simulink model "a2_clutch_control_sim"  (R2022b)
settings: Solver=VariableStepAuto  StartTime=0.0  StopTime=60  RelTol=1e-3
values from neighbouring files (symbols this model uses):
  Kd = 0.0033    [a1_performance_analysis_PD.m]    (also in a1_performance_analysis_PD_vs_Template.m; a2_hinf_control.m; a2_hinf_control_uncertainties.m)
  Kp = 0.3    [a1_performance_analysis_PD.m]    (also in a1_performance_analysis_PD_vs_Template.m; a2_hinf_control.m; a2_hinf_control_uncertainties.m)
  noise_fre = 800    [a2_hinf_control.m]    (also in a2_hinf_control_uncertainties.m)
undefined symbols (not defined in the file or in its folder): K_inf, vx
libraries: cstblocks x4, slpidlib x1
settings Model: Creator=phatdo  LastModifiedBy=phatdo
settings DataIOCC: ReturnWorkspaceOutputs=off

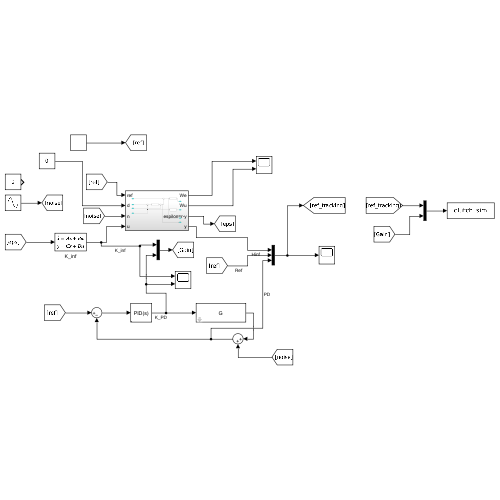
[thumbnail: Simulink's stored preview of the top-level diagram]
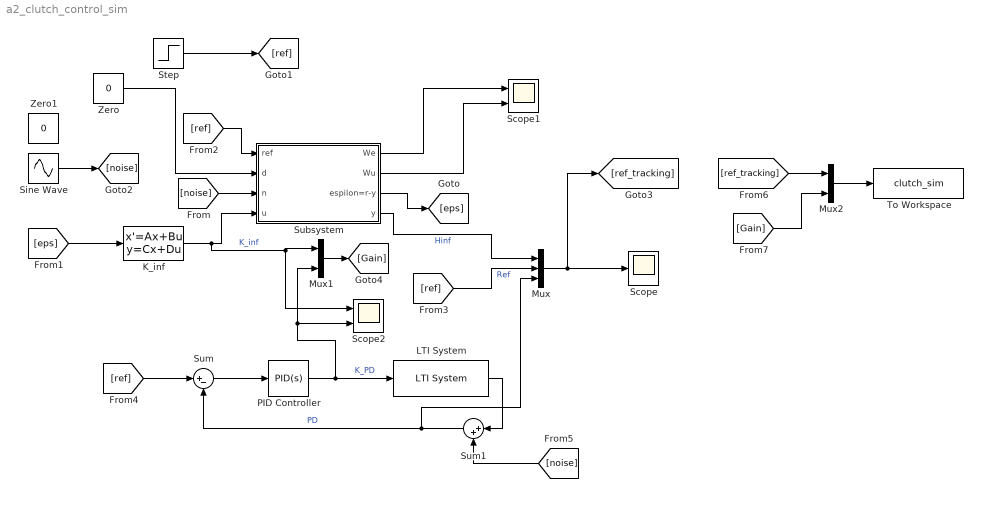
== system a2_clutch_control_sim ==
  K_inf : StateSpace  A=K_inf.A  B=K_inf.B  C=K_inf.C  D=K_inf.D  InitialCondition=[0]
  LTI System : cstblocks/LTI System  sys=G  IC=[vx]
  Mux : Mux  Inputs=3
  Mux1 : Mux  Inputs=2
  Mux2 : Mux  Inputs=2
  PID Controller : slpidlib/PID Controller  Controller=PID  Form=Parallel  TimeDomain=Continuous-time  UseExternalTs=off  SampleTime=-1  IntegratorMethod=Forward Euler  FilterMethod=Forward Euler  ControllerParametersSource=internal  P=Kp  I=1  UseKiTs=off  D=Kd  N=100  UseFilter=on  TunerSelectOption=Transfer Function Based (PID Tuner App)  InitialConditionSource=internal  InitialConditionForIntegrator=0  InitialConditionForFilter=0  DifferentiatorICPrevScaledInput=0  ExternalReset=none  TrackingMode=off  Kt=1  LimitOutput=off  SatLimitsSource=internal  UpperSaturationLimit=inf  LowerSaturationLimit=-inf  LinearizeAsGain=on  AntiWindupMode=none  Kb=1  LimitIntegrator=off  UpperIntegratorSaturationLimit=inf  LowerIntegratorSaturationLimit=-inf  POutMin=[]  POutMax=[]  IOutMin=[]  IOutMax=[]  DOutMin=[]  DOutMax=[]  NOutMin=[]  NOutMax=[]  SumOutMin=[]  SumOutMax=[]  SaturationOutMin=[]  SaturationOutMax=[]  PParamMin=[]  PParamMax=[]  IParamMin=[]  IParamMax=[]  DParamMin=[]  DParamMax=[]  NParamMin=[]  NParamMax=[]  KbParamMin=[]  KbParamMax=[]  KtParamMin=[]  KtParamMax=[]  KbOutMin=[]  KbOutMax=[]  KtOutMin=[]  KtOutMax=[]  IntegratorOutMin=[]  IntegratorOutMax=[]  FilterOutMin=[]  FilterOutMax=[]  SumI1OutMin=[]  SumI1OutMax=[]  SumI2OutMin=[]  SumI2OutMax=[]  SumI3OutMin=[]  SumI3OutMax=[]  SumI4OutMin=[]  SumI4OutMax=[]  SumDOutMin=[]  SumDOutMax=[]  DifferentiatorOutMin=[]  DifferentiatorOutMax=[]  FilterDiffOutCoefMin=[]  FilterDiffOutCoefMax=[]  ReciprocalOutMin=[]  ReciprocalOutMax=[]  SumDenOutMin=[]  SumDenOutMax=[]  SumNumOutMin=[]  SumNumOutMax=[]  DivideOutMin=[]  DivideOutMax=[]  UdiffTsProdOutMin=[]  UdiffTsProdOutMax=[]  NTsProdOutMin=[]  NTsProdOutMax=[]  UintegralTsProdOutMin=[]  UintegralTsProdOutMax=[]  UngainTsProdOutMin=[]  UngainTsProdOutMax=[]  ClampingZeroOutDataTypeStr=Inherit: Inherit via back propagation  ClampingZeroOutMin=[]  ClampingZeroOutMax=[]  FilterDenConstantOutDataTypeStr=Inherit: Inherit via back propagation  FilterDenConstantOutMin=[]  FilterDenConstantOutMax=[]  PCopyOutDataTypeStr=Inherit: Inherit via back propagation  PCopyOutMin=[]  PCopyOutMax=[]  NCopyOutDataTypeStr=Inherit: Inherit via back propagation  NCopyOutMin=[]  NCopyOutMax=[]  IntegratorContinuousStateAttributes=''  IntegratorStateMustResolveToSignalObject=off  IntegratorRTWStateStorageClass=Auto  FilterContinuousStateAttributes=''  FilterStateMustResolveToSignalObject=off  FilterRTWStateStorageClass=Auto  ParallelPVariant=InternalParameters  IdealPVariant=Disabled  IVariant=InternalParameters  DVariant=InternalParameters  IntegratorVariant=Continuous  SatVariant=Disabled  AWVariant=Passthrough  PCopyVariant=Disabled  TRVariant=Disabled  FdbkBlocksVariant=Forward  IdealPFdbkVariant=Disabled  SatFdbkVariant=Disabled  DerivativeFilterVariant=ContFilter  NVariant=InternalParameters  NCopyVariant=Disabled  FilterICVariant=InternalICsFilter  IntegratorICVariant=InternalICs  ExternalResetVariant=Disabled  TRSumVariant=Passthrough  SumFdbkVariant=Disabled  SumVariant=Sum_PID  TsampFilterVariant=InternalTs  TsampNgainVariant=Passthrough  TsampIntegralVariant=Passthrough  ExternalSaturationOutDataTypeStr=Inherit: Same as second input
  Scope : Scope
  Scope1 : Scope  NumInputPorts=2
  Scope2 : Scope  NumInputPorts=2
  Sine Wave : Sin  Amplitude=0.1  Frequency=noise_fre  SampleTime=0
  Step : Step  SampleTime=0
  Subsystem : Subsystem
  Sum : Sum  Inputs=|+-
  Sum1 : Sum  Inputs=|++
  To Workspace : ToWorkspace  VariableName=clutch_sim  SaveFormat=Timeseries  SampleTime=-1
  Zero : Constant  Value=0  OutDataTypeStr=Inherit: Inherit via back propagation
  Zero1 : Constant  Value=0  OutDataTypeStr=Inherit: Inherit via back propagation
  wires:
  Subsystem/1(We) -> Scope1/1
  Subsystem/2(Wu) -> Scope1/2
  Zero/1 -> Subsystem/2(d)
  K_inf/1 -> Scope2/1, Mux1/1, Subsystem/4(u)  "K_inf"
  Subsystem/3(espilon=r-y) -> [eps]
  [eps] -> K_inf/1
  Subsystem/4(y) -> Mux/1  "Hinf"
  Step/1 -> [ref]
  [ref] -> Subsystem/1(ref)
  [ref] -> Mux/2  "Ref"
  Mux/1 -> [ref_tracking], Scope/1
  LTI System/1 -> Sum1/1
  [ref] -> Sum/1
  Sum/1 -> PID Controller/1
  PID Controller/1 -> Mux1/2, Scope2/2, LTI System/1  "K_PD"
  Sum1/1 -> Mux/3, Sum/2  "PD"
  [noise] -> Subsystem/3(n)
  [noise] -> Sum1/2
  Mux1/1 -> [Gain]
  [ref_tracking] -> Mux2/1
  [Gain] -> Mux2/2
  Mux2/1 -> To Workspace/1
  Sine Wave/1 -> [noise]

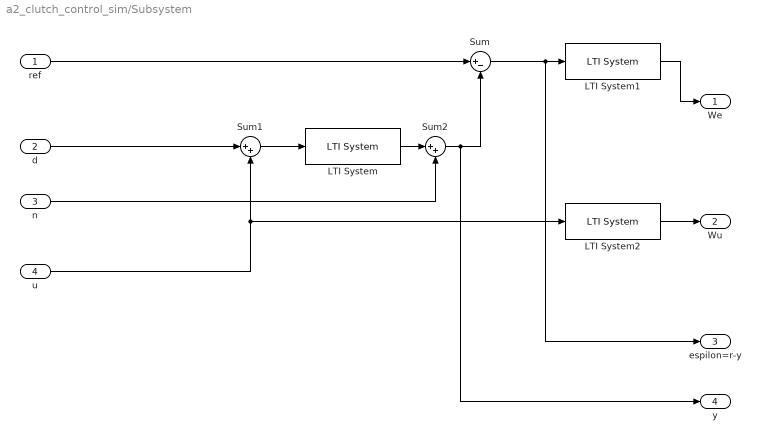
== system a2_clutch_control_sim/Subsystem ==
  ref : Inport  PortDimensions=1
  d : Inport  Port=2  PortDimensions=1
  n : Inport  Port=3  PortDimensions=1
  u : Inport  Port=4  PortDimensions=1
  LTI System : cstblocks/LTI System  sys=G  IC=[vx]
  LTI System1 : cstblocks/LTI System  sys=We  IC=[]
  LTI System2 : cstblocks/LTI System  sys=Wu  IC=[]
  Sum : Sum  Inputs=|+-
  Sum1 : Sum  Inputs=|++
  Sum2 : Sum  Inputs=|++
  We : Outport  PortDimensions=1  VectorParamsAs1DForOutWhenUnconnected=off
  Wu : Outport  Port=2  PortDimensions=1  VectorParamsAs1DForOutWhenUnconnected=off
  espilon=r-y : Outport  Port=3  PortDimensions=1  VectorParamsAs1DForOutWhenUnconnected=off
  y : Outport  Port=4  PortDimensions=1  VectorParamsAs1DForOutWhenUnconnected=off
  wires:
  LTI System2/1 -> Wu/1
  ref/1 -> Sum/1
  Sum/1 -> espilon=r-y/1, LTI System1/1
  u/1 -> Sum1/2, LTI System2/1
  LTI System1/1 -> We/1
  d/1 -> Sum1/1
  Sum1/1 -> LTI System/1
  LTI System/1 -> Sum2/1
  n/1 -> Sum2/2
  Sum2/1 -> y/1, Sum/2
